simulink model "WEEK1_QN9"  (R2020b)
settings: Solver=VariableStepAuto  StartTime=0.0  StopTime=10.0  RelTol=1e-3
model workspace (MAT data in the model file):
  B = 1e-06
  J = 1.517e-05
  Ke = 3.16333479321e-11
  L = 0.00505
  P = 4
  R = 4.98
  Sig = Simulink.Signal
  Sig.DataType = 'auto'
  Sig.Dimensions = -1
  Sig.DimensionsMode = 'auto'
  Sig.Complexity = 'auto'
  Sig.SampleTime = -1
  Sig.SamplingMode = 'auto'
  Sig1 = Simulink.Signal
  Sig1.DataType = 'auto'
  Sig1.Dimensions = -1
  Sig1.DimensionsMode = 'auto'
  Sig1.Complexity = 'auto'
  Sig1.SampleTime = -1
  Sig1.SamplingMode = 'auto'
  Tm = 0.1
  V = 30
  Va = 30
  Vb = 0
  Vc = 0
  w = 1
settings Model: Creator=dell  LastModifiedBy=dell

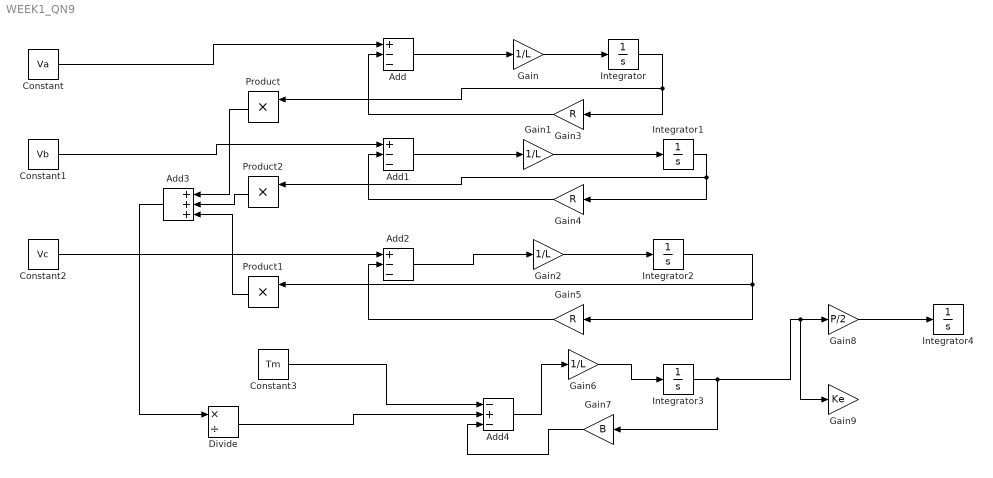
== system WEEK1_QN9 ==
  Add : Sum  Inputs=+--
  Add1 : Sum  Inputs=+--
  Add2 : Sum  Inputs=+--
  Add3 : Sum  Inputs=+++
  Add4 : Sum  Inputs=-+-
  Constant : Constant  Value=Va
  Constant1 : Constant  Value=Vb
  Constant2 : Constant  Value=Vc
  Constant3 : Constant  Value=Tm
  Divide : Product  Inputs=*/
  Gain{,1..2,6} (4 alike) : Gain  Gain=1/L
  Gain3 : Gain  Gain=R
  Gain4 : Gain  Gain=R
  Gain5 : Gain  Gain=R
  Gain7 : Gain  Gain=B
  Gain8 : Gain  Gain=P/2
  Gain9 : Gain  Gain=Ke
  Integrator{,1..4} (5 alike) : Integrator
  Product : Product
  Product1 : Product
  Product2 : Product
  wires:
  Add/1 -> Gain/1
  Gain/1 -> Integrator/1
  Integrator/1 -> Product/1, Gain3/1
  Gain3/1 -> Add/2
  Constant/1 -> Add/1
  Constant1/1 -> Add1/1
  Constant2/1 -> Add2/1
  Gain4/1 -> Add1/2
  Gain5/1 -> Add2/2
  Gain1/1 -> Integrator1/1
  Integrator1/1 -> Gain4/1, Product2/1
  Integrator2/1 -> Product1/1, Gain5/1
  Gain2/1 -> Integrator2/1
  Add2/1 -> Gain2/1
  Product/1 -> Add3/1
  Product2/1 -> Add3/2
  Product1/1 -> Add3/3
  Add1/1 -> Gain1/1
  Integrator3/1 -> Gain9/1, Gain8/1, Gain7/1
  Gain6/1 -> Integrator3/1
  Add4/1 -> Gain6/1
  Gain7/1 -> Add4/3
  Constant3/1 -> Add4/1
  Add3/1 -> Divide/1
  Divide/1 -> Add4/2
  Gain8/1 -> Integrator4/1
